simulink model "BFE_TestHarness"  (Simulink 8.6)
settings: Solver=FixedStepDiscrete  StartTime=0.0  StopTime=3  FixedStep=Ts  RelTol=1e-3
PreLoadFcn:
  | addpath('MBD_Tests')
  | 
  | load('Workspace\EnvVar.mat')
  | run('MBD_Tests\MBD_tests_init.m')
  | if exist('tl_preloadfcn','file'), tl_preloadfcn(gcs,402); end
PostLoadFcn:
  | if exist('tl_postloadfcn','file'), tl_postloadfcn(gcs,402); end
InitFcn:
  | if exist('tlds_init','file'), tlds_init(gcs); end
StartFcn:
  | if exist('tlds_start','file'), tlds_start(gcs); end
StopFcn:
  | if exist('tlds_stop','file'), tlds_stop(gcs); end
undefined symbols (not defined in the file): ddv, Ts, u2, u3, u4
libraries: tllib x11, simulink x8, LIB_TF_G_111 x2, LIB_TF_G_12_StepControl x2, LIB_TF_G_112 x1, LIB_TF_G_113 x1
(part 5 of 17)

== system BFE_TestHarness/BFE_AC_BeltFunctionExecution/Subsystem/BFE_AC_BeltFunctionExecution/BFE_AC_BeltFunctionExecution/ManageRunnables/If Action Subsystem2 ==
  PyroTriggeringStatus : Inport
  Trigger : TriggerPort  RequirementInfo={} %GIDa_866c371e_c2ef_4c5d_87b4_f06b2642b18c  TriggerType=function-call
  Constant : Constant  Value=170  mask(TL_Constant){data={'date',735951.66842896992}}
      settings: CopyFcn=if exist('tl_reset_reviewflag','file')==2,tl_reset_reviewflag(gcbh);end  DeleteFcn=if exist('delete_tlblock','file')==2,delete_tlblock(gcbh);end  NameChangeFcn=if exist('rename_tlblock','file')==2,rename_tlblock(gcbh);end  OpenFcn=if exist('tl_open_blockdlg','file')==2,tl_open_blockdlg(gcbh);else,open_system(gcbh,'parameter');end
      mask Help: eval(['if exist(''tl_online_help'',''file'') == 2, tl_online_help(''Topic'',''TL_Constant''),else, web([''jar:file:///'',matlabroot,''/help/toolbox/simulink/help.jar!/slref/' lower(get_param(gcbh,'Blocktype')) '.html''], ''-helpbrowser''),end'])
      mask Display: plot([-0.05, 1.05, NaN, -0.05, 1.05],[.01, .01, NaN, .99, .99])
  If Action Subsystem1 : Subsystem  RequirementInfo={} %GIDa_110f901d_19b3_4a41_884d_c39130871650  TreatAsAtomicUnit=on
  If Action Subsystem2 : Subsystem  RequirementInfo={} %GIDa_d22d9cd8_625f_49e4_bcfa_14ccc98dd57b  TreatAsAtomicUnit=on
  If1 : If  RequirementInfo={} %GIDa_090323af_991c_4502_8351_d7e3f5c13a0a  IfExpression=u1
  Relational Operator : RelationalOperator  Operator===  OutDataTypeStr=boolean  mask(TL_RelationalOperator){data={'date',735951.66842861113}}
      settings: DeleteFcn=if exist('delete_tlblock','file')==2,delete_tlblock(gcbh);end  NameChangeFcn=if exist('rename_tlblock','file')==2,rename_tlblock(gcbh);end  OpenFcn=if exist('tl_open_blockdlg','file')==2,tl_open_blockdlg(gcbh);else,open_system(gcbh,'parameter');end
      mask Help: eval(['if exist(''tl_online_help'',''file'') == 2, tl_online_help(''Topic'',''TL_RelationalOperator''),else, web([''jar:file:///'',matlabroot,''/help/toolbox/simulink/help.jar!/slref/' lower(get_param(gcbh,'Blocktype')) '.html''], ''-helpbrowser''),end'])
      mask Display: plot([-0.05, 1.05, NaN, -0.05, 1.05],[.01, .01, NaN, .99, .99])
  Out1 : Outport  RequirementInfo={} %GIDa_56619d25_d3d5_4dfa_b3ef_d6aa2f335483
  Out2 : Outport  RequirementInfo={} %GIDa_b3d42cdd_db79_4247_be88_47ad93015c12  Port=2
  wires:
  PyroTriggeringStatus/1 -> Relational Operator/2
  Constant/1 -> Relational Operator/1
  Relational Operator/1 -> If1/1
  If1/1 -> If Action Subsystem1/Action
  If Action Subsystem1/1(Out1) -> Out1/1
  If Action Subsystem2/1(Out1) -> Out2/1
  If1/2 -> If Action Subsystem2/Action

== system BFE_TestHarness/BFE_AC_BeltFunctionExecution/Subsystem/BFE_AC_BeltFunctionExecution/BFE_AC_BeltFunctionExecution/ManageRunnables/If Action Subsystem3 ==
  ResetMotorStageStatusRq : Inport
  Trigger : TriggerPort  RequirementInfo={} %GIDa_ecae3cd9_2f7e_4015_a246_5be66d2a3606  TriggerType=function-call
  Constant : Constant  Value=170  mask(TL_Constant){data={'date',735951.66842896992}}
      settings: CopyFcn=if exist('tl_reset_reviewflag','file')==2,tl_reset_reviewflag(gcbh);end  DeleteFcn=if exist('delete_tlblock','file')==2,delete_tlblock(gcbh);end  NameChangeFcn=if exist('rename_tlblock','file')==2,rename_tlblock(gcbh);end  OpenFcn=if exist('tl_open_blockdlg','file')==2,tl_open_blockdlg(gcbh);else,open_system(gcbh,'parameter');end
      mask Help: eval(['if exist(''tl_online_help'',''file'') == 2, tl_online_help(''Topic'',''TL_Constant''),else, web([''jar:file:///'',matlabroot,''/help/toolbox/simulink/help.jar!/slref/' lower(get_param(gcbh,'Blocktype')) '.html''], ''-helpbrowser''),end'])
      mask Display: plot([-0.05, 1.05, NaN, -0.05, 1.05],[.01, .01, NaN, .99, .99])
  If Action Subsystem1 : Subsystem  RequirementInfo={} %GIDa_dd934f85_730c_418a_8463_9eeb7f8d679a  TreatAsAtomicUnit=on
  If1 : If  RequirementInfo={} %GIDa_46faa83a_ad1e_4bf6_b8ac_9d2c86ced2b9  IfExpression=u1  ShowElse=off
  Relational Operator : RelationalOperator  Operator===  OutDataTypeStr=boolean  mask(TL_RelationalOperator){data={'date',735951.66842861113}}
      settings: DeleteFcn=if exist('delete_tlblock','file')==2,delete_tlblock(gcbh);end  NameChangeFcn=if exist('rename_tlblock','file')==2,rename_tlblock(gcbh);end  OpenFcn=if exist('tl_open_blockdlg','file')==2,tl_open_blockdlg(gcbh);else,open_system(gcbh,'parameter');end
      mask Help: eval(['if exist(''tl_online_help'',''file'') == 2, tl_online_help(''Topic'',''TL_RelationalOperator''),else, web([''jar:file:///'',matlabroot,''/help/toolbox/simulink/help.jar!/slref/' lower(get_param(gcbh,'Blocktype')) '.html''], ''-helpbrowser''),end'])
      mask Display: plot([-0.05, 1.05, NaN, -0.05, 1.05],[.01, .01, NaN, .99, .99])
  Out1 : Outport  RequirementInfo={} %GIDa_28cc5c12_1c46_425e_8111_f45bb80ffe30
  wires:
  ResetMotorStageStatusRq/1 -> Relational Operator/2
  Constant/1 -> Relational Operator/1
  Relational Operator/1 -> If1/1
  If1/1 -> If Action Subsystem1/Action
  If Action Subsystem1/1(Out1) -> Out1/1

== system BFE_TestHarness/BFE_AC_BeltFunctionExecution/Subsystem/BFE_AC_BeltFunctionExecution/BFE_AC_BeltFunctionExecution/BFE_runExecuteEmergencyBrakingSequence/ANG regulation/If Action Subsystem1 ==
  MotorPowerOrder : Inport  RequirementInfo={} %GIDa_36d63cdb_a1d7_45a0_bcbf_80961496797e  OutDataTypeStr=int16
  BoostPowerOrder : Inport  RequirementInfo={} %GIDa_d004899a_d052_4335_b4bf_8a07050271f2  Port=2  OutDataTypeStr=int16
  Action Port : ActionPort  RequirementInfo={} %GIDa_6a1bd9e6_01e7_4561_9119_4cca6ef02b4f  ActionType=then
  Data Store Write1 : DataStoreWrite  RequirementInfo={} %GIDa_807db9b2_3118_4ee1_b27d_6a192b350bd3  DataStoreName=BoostPowerOrder  mask(TL_DataStoreWrite){data={'date',735951.66861781245}}
      settings: DeleteFcn=if exist('delete_tlblock','file')==2,delete_tlblock(gcbh);end  NameChangeFcn=if exist('rename_tlblock','file')==2,rename_tlblock(gcbh);end  OpenFcn=if exist('tl_open_blockdlg','file')==2,tl_open_blockdlg(gcbh);else,open_system(gcbh,'parameter');end
      mask Help: eval(['if exist(''tl_online_help'',''file'') == 2, tl_online_help(''Topic'',''TL_DataStoreWrite''),else, web([''jar:file:///'',matlabroot,''/help/toolbox/simulink/help.jar!/slref/' lower(get_param(gcbh,'Blocktype')) '.html''], ''-helpbrowser''),end'])
      mask Display: plot([-0.05, 1.05, NaN, -0.05, 1.05],[.01, .01, NaN, .99, .99])
  Data Store Write2 : DataStoreWrite  RequirementInfo={} %GIDa_2a3ecfdf_d14c_4a9d_9b7c_c5a49fc3f0a5  DataStoreName=MotorPowerOrder  mask(TL_DataStoreWrite){data={'date',735951.6686177199}}
      settings: DeleteFcn=if exist('delete_tlblock','file')==2,delete_tlblock(gcbh);end  NameChangeFcn=if exist('rename_tlblock','file')==2,rename_tlblock(gcbh);end  OpenFcn=if exist('tl_open_blockdlg','file')==2,tl_open_blockdlg(gcbh);else,open_system(gcbh,'parameter');end
      mask Help: eval(['if exist(''tl_online_help'',''file'') == 2, tl_online_help(''Topic'',''TL_DataStoreWrite''),else, web([''jar:file:///'',matlabroot,''/help/toolbox/simulink/help.jar!/slref/' lower(get_param(gcbh,'Blocktype')) '.html''], ''-helpbrowser''),end'])
      mask Display: plot([-0.05, 1.05, NaN, -0.05, 1.05],[.01, .01, NaN, .99, .99])
  wires:
  MotorPowerOrder/1 -> Data Store Write2/1
  BoostPowerOrder/1 -> Data Store Write1/1

== system BFE_TestHarness/BFE_AC_BeltFunctionExecution/Subsystem/BFE_AC_BeltFunctionExecution/BFE_AC_BeltFunctionExecution/BFE_runExecuteEmergencyBrakingSequence/ANG regulation/Product ==
  In_1 : Inport
  In_2 : Inport  Port=2
  In_3 : Inport  Port=3
  Product : Product  Inputs=**  OutDataTypeStr=uint32  RndMeth=Zero  mask(TL_Product){data={'output',{'type','UInt32'},'date',735951.6686142477}}
      settings: CopyFcn=if exist('tl_reset_reviewflag','file')==2,tl_reset_reviewflag(gcbh);end  DeleteFcn=if exist('delete_tlblock','file')==2,delete_tlblock(gcbh);end  NameChangeFcn=if exist('rename_tlblock','file')==2,rename_tlblock(gcbh);end  OpenFcn=if exist('tl_open_blockdlg','file')==2,tl_open_blockdlg(gcbh);else,open_system(gcbh,'parameter');end
      mask Help: eval(['if exist(''tl_online_help'',''file'') == 2, tl_online_help(''Topic'',''TL_Product''),else, web([''jar:file:///'',matlabroot,''/help/toolbox/simulink/help.jar!/slref/' lower(get_param(gcbh,'Blocktype')) '.html''], ''-helpbrowser''),end'])
      mask Display: plot([-0.05, 1.05, NaN, -0.05, 1.05],[.01, .01, NaN, .99, .99])
  Product_1 : Product  Inputs=**  RndMeth=Zero  mask(TL_Product){data={'output',{'type','UInt32'},'date',735951.66861386574}}
      settings: CopyFcn=if exist('tl_reset_reviewflag','file')==2,tl_reset_reviewflag(gcbh);end  DeleteFcn=if exist('delete_tlblock','file')==2,delete_tlblock(gcbh);end  NameChangeFcn=if exist('rename_tlblock','file')==2,rename_tlblock(gcbh);end  OpenFcn=if exist('tl_open_blockdlg','file')==2,tl_open_blockdlg(gcbh);else,open_system(gcbh,'parameter');end
      mask Help: eval(['if exist(''tl_online_help'',''file'') == 2, tl_online_help(''Topic'',''TL_Product''),else, web([''jar:file:///'',matlabroot,''/help/toolbox/simulink/help.jar!/slref/' lower(get_param(gcbh,'Blocktype')) '.html''], ''-helpbrowser''),end'])
      mask Display: plot([-0.05, 1.05, NaN, -0.05, 1.05],[.01, .01, NaN, .99, .99])
  Out_1 : Outport
  wires:
  In_1/1 -> Product_1/1
  In_2/1 -> Product_1/2
  In_3/1 -> Product/2
  Product_1/1 -> Product/1
  Product/1 -> Out_1/1

== system BFE_TestHarness/BFE_AC_BeltFunctionExecution/Subsystem/BFE_AC_BeltFunctionExecution/BFE_AC_BeltFunctionExecution/BFE_runExecuteEmergencyBrakingSequence/ANG regulation/Src ==
  Const : Constant  Value=ddv('RTE_Define/KU8_MOTOR_STAGE_EMERGENCY_DEACTIVATION')  mask(TL_Constant){data={'output',{'variable','RTE_Define/KU8_MOTOR_STAGE_EMERGENCY_DEACTIVATION'},'date',735951.66861100693}}
      settings: CopyFcn=if exist('tl_reset_reviewflag','file')==2,tl_reset_reviewflag(gcbh);end  DeleteFcn=if exist('delete_tlblock','file')==2,delete_tlblock(gcbh);end  NameChangeFcn=if exist('rename_tlblock','file')==2,rename_tlblock(gcbh);end  OpenFcn=if exist('tl_open_blockdlg','file')==2,tl_open_blockdlg(gcbh);else,open_system(gcbh,'parameter');end
      mask Help: eval(['if exist(''tl_online_help'',''file'') == 2, tl_online_help(''Topic'',''TL_Constant''),else, web([''jar:file:///'',matlabroot,''/help/toolbox/simulink/help.jar!/slref/' lower(get_param(gcbh,'Blocktype')) '.html''], ''-helpbrowser''),end'])
      mask Display: plot([-0.05, 1.05, NaN, -0.05, 1.05],[.01, .01, NaN, .99, .99])
  u8MotorStageStatus : Outport
  wires:
  Const/1 -> u8MotorStageStatus/1  "u8MotorStageStatus"

== system BFE_TestHarness/BFE_AC_BeltFunctionExecution/Subsystem/BFE_AC_BeltFunctionExecution/BFE_AC_BeltFunctionExecution/BFE_runExecuteEmergencyBrakingSequence/Idle State/If Action Subsystem ==
  MotorPowerOrder : Inport  RequirementInfo={} %GIDa_39707416_cbd7_49a4_89b1_309ad3050f45  OutDataTypeStr=int16
  BoostPowerOrder : Inport  RequirementInfo={} %GIDa_de3b3d4e_919a_4afc_a9bd_d52a78375d81  Port=2  OutDataTypeStr=int16
  Action Port : ActionPort  RequirementInfo={} %GIDa_e9528953_7f61_49b7_b615_23fe905f704f  ActionType=then
  Data Store Write1 : DataStoreWrite  RequirementInfo={} %GIDa_59c6ee34_e957_4309_9132_375d2670ef26  DataStoreName=BoostPowerOrder  mask(TL_DataStoreWrite){data={'date',735951.66860575229}}
      settings: DeleteFcn=if exist('delete_tlblock','file')==2,delete_tlblock(gcbh);end  NameChangeFcn=if exist('rename_tlblock','file')==2,rename_tlblock(gcbh);end  OpenFcn=if exist('tl_open_blockdlg','file')==2,tl_open_blockdlg(gcbh);else,open_system(gcbh,'parameter');end
      mask Help: eval(['if exist(''tl_online_help'',''file'') == 2, tl_online_help(''Topic'',''TL_DataStoreWrite''),else, web([''jar:file:///'',matlabroot,''/help/toolbox/simulink/help.jar!/slref/' lower(get_param(gcbh,'Blocktype')) '.html''], ''-helpbrowser''),end'])
      mask Display: plot([-0.05, 1.05, NaN, -0.05, 1.05],[.01, .01, NaN, .99, .99])
  Data Store Write2 : DataStoreWrite  RequirementInfo={} %GIDa_3b8346d3_29b2_4ee4_8164_42224b922a82  DataStoreName=MotorPowerOrder  mask(TL_DataStoreWrite){data={'date',735951.6686056481}}
      settings: DeleteFcn=if exist('delete_tlblock','file')==2,delete_tlblock(gcbh);end  NameChangeFcn=if exist('rename_tlblock','file')==2,rename_tlblock(gcbh);end  OpenFcn=if exist('tl_open_blockdlg','file')==2,tl_open_blockdlg(gcbh);else,open_system(gcbh,'parameter');end
      mask Help: eval(['if exist(''tl_online_help'',''file'') == 2, tl_online_help(''Topic'',''TL_DataStoreWrite''),else, web([''jar:file:///'',matlabroot,''/help/toolbox/simulink/help.jar!/slref/' lower(get_param(gcbh,'Blocktype')) '.html''], ''-helpbrowser''),end'])
      mask Display: plot([-0.05, 1.05, NaN, -0.05, 1.05],[.01, .01, NaN, .99, .99])
  wires:
  MotorPowerOrder/1 -> Data Store Write2/1
  BoostPowerOrder/1 -> Data Store Write1/1

== system BFE_TestHarness/BFE_AC_BeltFunctionExecution/Subsystem/BFE_AC_BeltFunctionExecution/BFE_AC_BeltFunctionExecution/BFE_runExecuteEmergencyBrakingSequence/Idle State/Src ==
  Const : Constant  Value=ddv('RTE_Define/KU8_MOTOR_STAGE_EMERGENCY_DEACTIVATION')  mask(TL_Constant){data={'output',{'variable','RTE_Define/KU8_MOTOR_STAGE_EMERGENCY_DEACTIVATION'},'date',735951.66860392364}}
      settings: CopyFcn=if exist('tl_reset_reviewflag','file')==2,tl_reset_reviewflag(gcbh);end  DeleteFcn=if exist('delete_tlblock','file')==2,delete_tlblock(gcbh);end  NameChangeFcn=if exist('rename_tlblock','file')==2,rename_tlblock(gcbh);end  OpenFcn=if exist('tl_open_blockdlg','file')==2,tl_open_blockdlg(gcbh);else,open_system(gcbh,'parameter');end
      mask Help: eval(['if exist(''tl_online_help'',''file'') == 2, tl_online_help(''Topic'',''TL_Constant''),else, web([''jar:file:///'',matlabroot,''/help/toolbox/simulink/help.jar!/slref/' lower(get_param(gcbh,'Blocktype')) '.html''], ''-helpbrowser''),end'])
      mask Display: plot([-0.05, 1.05, NaN, -0.05, 1.05],[.01, .01, NaN, .99, .99])
  u8MotorStageStatus : Outport
  wires:
  Const/1 -> u8MotorStageStatus/1  "u8MotorStageStatus"

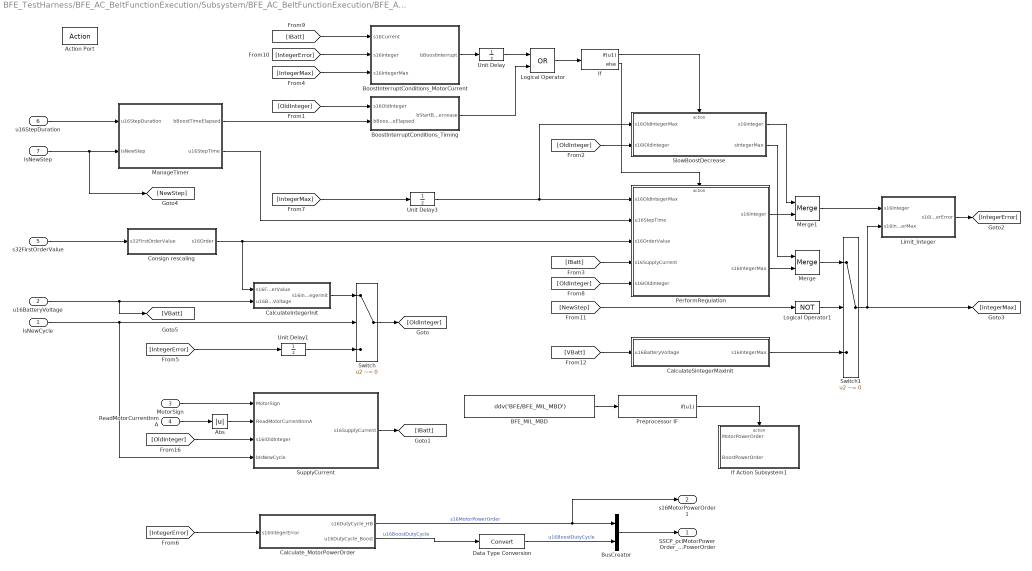
== system BFE_TestHarness/BFE_AC_BeltFunctionExecution/Subsystem/BFE_AC_BeltFunctionExecution/BFE_AC_BeltFunctionExecution/BFE_runExecuteHighPowerStep/HP feature activated/CurrentRegulation ==
  IsNewCycle : Inport  RequirementInfo={} %GIDa_1662e31c_4847_435c_863a_1ec5eca2756d
  u16BatteryVoltage : Inport  RequirementInfo={} %GIDa_1bb34935_6dbf_432a_9b43_0281e74792fd  Port=2
  MotorSign : Inport  RequirementInfo={} %GIDa_5fb47f80_c22b_46b0_b1d3_660182323a24  Port=3
  ReadMotorCurrentInmA : Inport  RequirementInfo={} %GIDa_31f7513d_9132_45be_9a79_4368bb0828a9  Port=4
  s32FirstOrderValue : Inport  RequirementInfo={} %GIDa_e04d25b8_d427_4e8e_8f00_3b1e8e5fec68  Port=5
  u16StepDuration : Inport  RequirementInfo={} %GIDa_4dbadef5_81a2_48d0_a2ca_74b2fd0262db  Port=6  OutDataTypeStr=uint16
  IsNewStep : Inport  RequirementInfo={} %GIDa_223ba4e3_ba54_41a4_96d0_22f7bdf9d99f  Port=7
  Action Port : ActionPort  RequirementInfo={} %GIDa_dfa5435c_c4b1_4a26_8b12_c66635d4e3dc  ActionType=then
  Abs : Abs  mask(TL_Abs){data={'output',{'type','UInt32'},'date',735951.66858795134}}
      settings: CopyFcn=if exist('tl_reset_reviewflag','file')==2,tl_reset_reviewflag(gcbh);end  DeleteFcn=if exist('delete_tlblock','file')==2,delete_tlblock(gcbh);end  NameChangeFcn=if exist('rename_tlblock','file')==2,rename_tlblock(gcbh);end  OpenFcn=if exist('tl_open_blockdlg','file')==2,tl_open_blockdlg(gcbh);else,open_system(gcbh,'parameter');end
      mask Help: eval(['if exist(''tl_online_help'',''file'') == 2, tl_online_help(''Topic'',''TL_Abs''),else, web([''jar:file:///'',matlabroot,''/help/toolbox/simulink/help.jar!/slref/' lower(get_param(gcbh,'Blocktype')) '.html''], ''-helpbrowser''),end'])
      mask Display: plot([-0.05, 1.05, NaN, -0.05, 1.05],[.01, .01, NaN, .99, .99])
  BFE_MIL_MBD : Constant  RequirementInfo={} %GIDa_b0161e3c_e162_4059_a91d_45f997bd6b1e  Value=ddv('BFE/BFE_MIL_MBD')  mask(TL_Constant){data={'output',{'variable','BFE/BFE_MIL_MBD'},'date',735951.66858758102}}
      settings: CopyFcn=if exist('tl_reset_reviewflag','file')==2,tl_reset_reviewflag(gcbh);end  DeleteFcn=if exist('delete_tlblock','file')==2,delete_tlblock(gcbh);end  NameChangeFcn=if exist('rename_tlblock','file')==2,rename_tlblock(gcbh);end  OpenFcn=if exist('tl_open_blockdlg','file')==2,tl_open_blockdlg(gcbh);else,open_system(gcbh,'parameter');end
      mask Help: eval(['if exist(''tl_online_help'',''file'') == 2, tl_online_help(''Topic'',''TL_Constant''),else, web([''jar:file:///'',matlabroot,''/help/toolbox/simulink/help.jar!/slref/' lower(get_param(gcbh,'Blocktype')) '.html''], ''-helpbrowser''),end'])
      mask Display: plot([-0.05, 1.05, NaN, -0.05, 1.05],[.01, .01, NaN, .99, .99])
  BoostInterruptConditions_MotorCurrent : Subsystem  RequirementInfo={} %GIDa_1e154413_408a_4156_80c5_1742329dab2b
  BoostInterruptConditions_Timing : Subsystem  RequirementInfo={} %GIDa_8282939d_02dc_455b_ba62_25a73597f55d
  BusCreator : BusCreator  Inputs=2
  CalculateIntegerInit : Subsystem  RequirementInfo={} %GIDa_9a2c8a86_eea1_4d27_b0ce_971bbb33bd14
  CalculateSintegerMaxInit : Subsystem  RequirementInfo={} %GIDa_66e9dbb1_52b6_4aae_afa6_381740208472  TreatAsAtomicUnit=on
  Calculate_MotorPowerOrder : Subsystem  RequirementInfo={} %GIDa_f695fff8_9d75_4e11_9ea4_5644486dca77
  Consign rescaling : Subsystem  TreatAsAtomicUnit=on
      settings: AttributesFormatString=8092 lsb = 0.5 [A]\nV\n1 lsb = 10 [mA]
  Data Type Conversion : DataTypeConversion
  If : If  RequirementInfo={} %GIDa_93686889_67cf_4afb_8e2f_6a5e4d238abf  IfExpression=u1
  If Action Subsystem1 : Subsystem  RequirementInfo={} %GIDa_73714641_df61_49fe_9fdd_bd97cd5bece8  TreatAsAtomicUnit=on
  Limit_Integer : Subsystem  RequirementInfo={} %GIDa_70b31615_98db_428c_aa79_8c8fa2e5a701
  Logical Operator : Logic  RequirementInfo={} %GIDa_fe6e0a6b_febe_46e6_a7cb_d3961de08f42  Operator=OR  AllPortsSameDT=off  OutDataTypeStr=boolean  mask(TL_LogicalOperator){data={'date',735951.66856991895}}
      settings: DeleteFcn=if exist('delete_tlblock','file')==2,delete_tlblock(gcbh);end  NameChangeFcn=if exist('rename_tlblock','file')==2,rename_tlblock(gcbh);end  OpenFcn=if exist('tl_open_blockdlg','file')==2,tl_open_blockdlg(gcbh);else,open_system(gcbh,'parameter');end
      mask Help: eval(['if exist(''tl_online_help'',''file'') == 2, tl_online_help(''Topic'',''TL_LogicalOperator''),else, web([''jar:file:///'',matlabroot,''/help/toolbox/simulink/help.jar!/slref/' lower(get_param(gcbh,'Blocktype')) '.html''], ''-helpbrowser''),end'])
      mask Display: plot([-0.05, 1.05, NaN, -0.05, 1.05],[.01, .01, NaN, .99, .99])
  Logical Operator1 : Logic  Operator=NOT  Inputs=1  AllPortsSameDT=off  OutDataTypeStr=boolean  mask(TL_LogicalOperator){data={'date',735951.66856965283}}
      settings: DeleteFcn=if exist('delete_tlblock','file')==2,delete_tlblock(gcbh);end  NameChangeFcn=if exist('rename_tlblock','file')==2,rename_tlblock(gcbh);end  OpenFcn=if exist('tl_open_blockdlg','file')==2,tl_open_blockdlg(gcbh);else,open_system(gcbh,'parameter');end
      mask Help: eval(['if exist(''tl_online_help'',''file'') == 2, tl_online_help(''Topic'',''TL_LogicalOperator''),else, web([''jar:file:///'',matlabroot,''/help/toolbox/simulink/help.jar!/slref/' lower(get_param(gcbh,'Blocktype')) '.html''], ''-helpbrowser''),end'])
      mask Display: plot([-0.05, 1.05, NaN, -0.05, 1.05],[.01, .01, NaN, .99, .99])
  ManageTimer : Subsystem  RequirementInfo={} %GIDa_aa7b4bf5_2b52_4aaf_8bb3_ae9b1da1e681
  Merge : Merge  RequirementInfo={} %GIDa_abd3f291_8f58_447c_99f5_868d95eb83d7  InitialOutput=0  mask(TL_Merge){data={'output',{'name','s16IntegerMaxOnGoing'},'date',735951.66844865738}}
      settings: CopyFcn=if exist('tl_reset_reviewflag','file')==2,tl_reset_reviewflag(gcbh);end  DeleteFcn=if exist('delete_tlblock','file')==2,delete_tlblock(gcbh);end  NameChangeFcn=if exist('rename_tlblock','file')==2,rename_tlblock(gcbh);end  OpenFcn=if exist('tl_open_blockdlg','file')==2,tl_open_blockdlg(gcbh);else,open_system(gcbh,'parameter');end
      mask Help: eval(['if exist(''tl_online_help'',''file'') == 2, tl_online_help(''Topic'',''TL_Merge''),else, web([''jar:file:///'',matlabroot,''/help/toolbox/simulink/help.jar!/slref/' lower(get_param(gcbh,'Blocktype')) '.html''], ''-helpbrowser''),end'])
      mask Display: plot([-0.05, 1.05, NaN, -0.05, 1.05],[.01, .01, NaN, .99, .99])
  Merge1 : Merge  RequirementInfo={} %GIDa_8234cb0a_dc3c_4713_a3c9_c2ddd3d4af5c  InitialOutput=0  mask(TL_Merge){data={'output',{'name','s16Integer'},'date',735951.66844827542}}
      settings: CopyFcn=if exist('tl_reset_reviewflag','file')==2,tl_reset_reviewflag(gcbh);end  DeleteFcn=if exist('delete_tlblock','file')==2,delete_tlblock(gcbh);end  NameChangeFcn=if exist('rename_tlblock','file')==2,rename_tlblock(gcbh);end  OpenFcn=if exist('tl_open_blockdlg','file')==2,tl_open_blockdlg(gcbh);else,open_system(gcbh,'parameter');end
      mask Help: eval(['if exist(''tl_online_help'',''file'') == 2, tl_online_help(''Topic'',''TL_Merge''),else, web([''jar:file:///'',matlabroot,''/help/toolbox/simulink/help.jar!/slref/' lower(get_param(gcbh,'Blocktype')) '.html''], ''-helpbrowser''),end'])
      mask Display: plot([-0.05, 1.05, NaN, -0.05, 1.05],[.01, .01, NaN, .99, .99])
  PerformRegulation : Subsystem  RequirementInfo={} %GIDa_1363a116_a98c_4e77_a913_b87844d45823
  Preprocessor IF : If  RequirementInfo={} %GIDa_f50148b4_caa7_4fb8_ad64_c4c8bcffd358  IfExpression=u1  ShowElse=off  mask(TL_PreProcessorIf){data={'mode',2,'date',735951.66844163195}}
      settings: DeleteFcn=if exist('delete_tlblock','file')==2,delete_tlblock(gcbh);end  NameChangeFcn=if exist('rename_tlblock','file')==2,rename_tlblock(gcbh);end  OpenFcn=if exist('tl_open_blockdlg','file')==2,tl_open_blockdlg(gcbh);else,open_system(gcbh,'parameter');end
      mask Help: eval(['if exist(''tl_online_help'',''file'') == 2, tl_online_help(''Topic'',''TL_PreProcessorIf''),else, web([''jar:file:///'',matlabroot,''/help/toolbox/simulink/help.jar!/slref/' lower(get_param(gcbh,'Blocktype')) '.html''], ''-helpbrowser''),end'])
      mask Display:
      | plot([-0.05, 1.05, NaN, -0.05, 1.05],[.01, .01, NaN, .99, .99])
      | 
      | port_label('input', 1, 'u1')
      | port_label('output',1,'#ifdef u1');
  SlowBoostDecrease : Subsystem  RequirementInfo={} %GIDa_3dda9a5c_4141_4318_8fb6_6c48e8effe73
  SupplyCurrent : Subsystem  TreatAsAtomicUnit=on
  Switch : Switch  RequirementInfo={} %GIDa_30553cb4_fd4d_48f0_a467_0ca3f5a035ff  Criteria=u2 ~= 0  mask(TL_Switch){data={'output',{'name','s16OldIntegerError'},'date',735951.66841892363}}
      settings: CopyFcn=if exist('tl_reset_reviewflag','file')==2,tl_reset_reviewflag(gcbh);end  DeleteFcn=if exist('delete_tlblock','file')==2,delete_tlblock(gcbh);end  NameChangeFcn=if exist('rename_tlblock','file')==2,rename_tlblock(gcbh);end  OpenFcn=if exist('tl_open_blockdlg','file')==2,tl_open_blockdlg(gcbh);else,open_system(gcbh,'parameter');end
      mask Help: eval(['if exist(''tl_online_help'',''file'') == 2, tl_online_help(''Topic'',''TL_Switch''),else, web([''jar:file:///'',matlabroot,''/help/toolbox/simulink/help.jar!/slref/' lower(get_param(gcbh,'Blocktype')) '.html''], ''-helpbrowser''),end'])
      mask Display: plot([-0.05, 1.05, NaN, -0.05, 1.05],[.01, .01, NaN, .99, .99])
  Switch1 : Switch  Criteria=u2 ~= 0  mask(TL_Switch){data={'output',{'name','s16IntegerMax'},'date',735951.66841839126}}
      settings: CopyFcn=if exist('tl_reset_reviewflag','file')==2,tl_reset_reviewflag(gcbh);end  DeleteFcn=if exist('delete_tlblock','file')==2,delete_tlblock(gcbh);end  NameChangeFcn=if exist('rename_tlblock','file')==2,rename_tlblock(gcbh);end  OpenFcn=if exist('tl_open_blockdlg','file')==2,tl_open_blockdlg(gcbh);else,open_system(gcbh,'parameter');end
      mask Help: eval(['if exist(''tl_online_help'',''file'') == 2, tl_online_help(''Topic'',''TL_Switch''),else, web([''jar:file:///'',matlabroot,''/help/toolbox/simulink/help.jar!/slref/' lower(get_param(gcbh,'Blocktype')) '.html''], ''-helpbrowser''),end'])
      mask Display: plot([-0.05, 1.05, NaN, -0.05, 1.05],[.01, .01, NaN, .99, .99])
  Unit Delay : UnitDelay  RequirementInfo={} %GIDa_40b8b31e_7c77_49f4_a8c4_1aef21ac2334  SampleTime=-1  mask(TL_UnitDelay){data={'state',{'name','bOldBoostInterrupt'},'date',735951.66841787042}}
      settings: CopyFcn=if exist('tl_reset_reviewflag','file')==2,tl_reset_reviewflag(gcbh);end  DeleteFcn=if exist('delete_tlblock','file')==2,delete_tlblock(gcbh);end  NameChangeFcn=if exist('rename_tlblock','file')==2,rename_tlblock(gcbh);end  OpenFcn=if exist('tl_open_blockdlg','file')==2,tl_open_blockdlg(gcbh);else,open_system(gcbh,'parameter');end
      mask Help: eval(['if exist(''tl_online_help'',''file'') == 2, tl_online_help(''Topic'',''TL_UnitDelay''),else, web([''jar:file:///'',matlabroot,''/help/toolbox/simulink/help.jar!/slref/' lower(get_param(gcbh,'Blocktype')) '.html''], ''-helpbrowser''),end'])
      mask Display: plot([-0.05, 1.05, NaN, -0.05, 1.05],[.01, .01, NaN, .99, .99])
  Unit Delay1 : UnitDelay  RequirementInfo={} %GIDa_fff37aa9_a0a1_4cec_b06f_6507d85e68da  SampleTime=-1  mask(TL_UnitDelay){data={'state',{'name','s16_OldIntegerError'},'date',735951.66841733793}}
      settings: CopyFcn=if exist('tl_reset_reviewflag','file')==2,tl_reset_reviewflag(gcbh);end  DeleteFcn=if exist('delete_tlblock','file')==2,delete_tlblock(gcbh);end  NameChangeFcn=if exist('rename_tlblock','file')==2,rename_tlblock(gcbh);end  OpenFcn=if exist('tl_open_blockdlg','file')==2,tl_open_blockdlg(gcbh);else,open_system(gcbh,'parameter');end
      mask Help: eval(['if exist(''tl_online_help'',''file'') == 2, tl_online_help(''Topic'',''TL_UnitDelay''),else, web([''jar:file:///'',matlabroot,''/help/toolbox/simulink/help.jar!/slref/' lower(get_param(gcbh,'Blocktype')) '.html''], ''-helpbrowser''),end'])
      mask Display: plot([-0.05, 1.05, NaN, -0.05, 1.05],[.01, .01, NaN, .99, .99])
  Unit Delay3 : UnitDelay  RequirementInfo={} %GIDa_408d93ed_0585_4d91_8b20_90bf83d81e20  SampleTime=-1  mask(TL_UnitDelay){data={'state',{'name','s16OldIntegerMax'},'date',735951.66841681709}}
      settings: CopyFcn=if exist('tl_reset_reviewflag','file')==2,tl_reset_reviewflag(gcbh);end  DeleteFcn=if exist('delete_tlblock','file')==2,delete_tlblock(gcbh);end  NameChangeFcn=if exist('rename_tlblock','file')==2,rename_tlblock(gcbh);end  OpenFcn=if exist('tl_open_blockdlg','file')==2,tl_open_blockdlg(gcbh);else,open_system(gcbh,'parameter');end
      mask Help: eval(['if exist(''tl_online_help'',''file'') == 2, tl_online_help(''Topic'',''TL_UnitDelay''),else, web([''jar:file:///'',matlabroot,''/help/toolbox/simulink/help.jar!/slref/' lower(get_param(gcbh,'Blocktype')) '.html''], ''-helpbrowser''),end'])
      mask Display: plot([-0.05, 1.05, NaN, -0.05, 1.05],[.01, .01, NaN, .99, .99])
  SSCP_pclMotorPowerOrder_SetPowerOrder : Outport  mask(TL_BusOutport){data={'#autoscaling',2,'#message',2,'#output',2,'#logdata',2,'signals',{{'',{'s16MotorPowerOrder';'u16BoostDutyCycle'}}},'autosar',{'useautosarcommunication',1,'kind',4,'clientserverport','pclMotor_P','operation','SetPowerOrder'},'date',736301.7172136805}}
      settings: CopyFcn=if exist('tl_reset_reviewflag','file')==2,tl_reset_reviewflag(gcbh);end  DeleteFcn=if exist('delete_tlblock','file')==2,delete_tlblock(gcbh);end  NameChangeFcn=if exist('rename_tlblock','file')==2,rename_tlblock(gcbh);end  OpenFcn=if exist('tl_open_blockdlg','file')==2,tl_open_blockdlg(gcbh);else,open_system(gcbh,'parameter');end
      mask Help: eval(['if exist(''tl_online_help'',''file'') == 2, tl_online_help(''Topic'',''TL_Outport''),else, web([''jar:file:///'',matlabroot,''/help/toolbox/simulink/help.jar!/slref/' lower(get_param(gcbh,'Blocktype')) '.html''], ''-helpbrowser''),end'])
      mask Display: plot([0.2 0.35 NaN 0.65 0.8],[0 1 NaN 0 1]);
  s16MotorPowerOrder1 : Outport  Port=2  PortDimensions=1  InitialOutput=0  mask(TL_Outport){data={'autosar',{'useautosarcommunication',1,'kind',3,'communicationmode',1,'interrunnablevariable','s16MotorPowerOrder'},'date',736809.44014787034}}
      settings: CopyFcn=if exist('tl_reset_reviewflag','file')==2,tl_reset_reviewflag(gcbh);end  DeleteFcn=if exist('delete_tlblock','file')==2,delete_tlblock(gcbh);end  NameChangeFcn=if exist('rename_tlblock','file')==2,rename_tlblock(gcbh);end  OpenFcn=if exist('tl_open_blockdlg','file')==2,tl_open_blockdlg(gcbh);else,open_system(gcbh,'parameter');end
      mask Help: eval(['if exist(''tl_online_help'',''file'') == 2, tl_online_help(''Topic'',''TL_Outport''),else, web([''jar:file:///'',matlabroot,''/help/toolbox/simulink/help.jar!/slref/' lower(get_param(gcbh,'Blocktype')) '.html''], ''-helpbrowser''),end'])
      mask Display: plot([0.2 0.35 NaN 0.65 0.8],[0 1 NaN 0 1]);
  wires:
  If/1 -> SlowBoostDecrease/Action
  If/2 -> PerformRegulation/Action
  s32FirstOrderValue/1 -> Consign rescaling/1(s32FirstOrderValue)
  IsNewStep/1 -> ManageTimer/2(IsNewStep), [NewStep]
  u16StepDuration/1 -> ManageTimer/1(u16StepDuration)
  SlowBoostDecrease/2(sIntegerMax) -> Merge/1
  PerformRegulation/1(s16Integer) -> Merge1/2
  CalculateIntegerInit/1(s16IntegerInit) -> Switch/1
  Unit Delay1/1 -> Switch/3
  SlowBoostDecrease/1(s16Integer) -> Merge1/1
  MotorSign/1 -> SupplyCurrent/1(MotorSign)
  ReadMotorCurrentInmA/1 -> Abs/1
  IsNewCycle/1 -> Switch/2, SupplyCurrent/4(bIsNewCycle)
  Logical Operator/1 -> If/1
  PerformRegulation/2(s16IntegerMax) -> Merge/2
  ManageTimer/1(bBoostTimeElapsed) -> BoostInterruptConditions_Timing/2(bBoostTimeElapsed)
  BoostInterruptConditions_Timing/1(bStartBoostDecrease) -> Logical Operator/2
  Switch/1 -> [OldInteger]
  [OldInteger] -> BoostInterruptConditions_Timing/1(s16OldInteger)
  [OldInteger] -> SlowBoostDecrease/2(s16IOldInteger)
  Unit Delay/1 -> Logical Operator/1
  SupplyCurrent/1(s16SupplyCurrent) -> [IBatt]
  [IBatt] -> PerformRegulation/4(s16SupplyCurrent)
  [IntegerError] -> Unit Delay1/1
  [OldInteger] -> PerformRegulation/5(s16IOldInteger)
  [IBatt] -> BoostInterruptConditions_MotorCurrent/1(s16Current)
  [IntegerError] -> BoostInterruptConditions_MotorCurrent/2(s16Integer)
  BoostInterruptConditions_MotorCurrent/1(bBoostInterrupt) -> Unit Delay/1
  Consign rescaling/1(s16Order) -> PerformRegulation/3(s16OrderValue), CalculateIntegerInit/1(s16FirstOrderValue)
  Unit Delay3/1 -> SlowBoostDecrease/1(s16OldIntegerMax), PerformRegulation/1(s16OldIntegerMax)
  [IntegerMax] -> BoostInterruptConditions_MotorCurrent/3(s16IntegerMax)
  [IntegerMax] -> Unit Delay3/1
  u16BatteryVoltage/1 -> CalculateIntegerInit/2(u16BatteryVoltage), [VBatt]
  Merge/1 -> Switch1/1
  CalculateSintegerMaxInit/1(s16IntegerMax) -> Switch1/3
  Switch1/1 -> Limit_Integer/2(s16IntegerMax), [IntegerMax]
  [NewStep] -> Logical Operator1/1
  Logical Operator1/1 -> Switch1/2
  [VBatt] -> CalculateSintegerMaxInit/1(u16BatteryVoltage)
  [OldInteger] -> SupplyCurrent/3(s16IOldInteger)
  Calculate_MotorPowerOrder/1(s16DutyCycle_HB) -> BusCreator/1, s16MotorPowerOrder1/1  "s16MotorPowerOrder"
  Calculate_MotorPowerOrder/2(u16DutyCycle_Boost) -> Data Type Conversion/1  "u16BoostDutyCycle"
  BusCreator/1 -> SSCP_pclMotorPowerOrder_SetPowerOrder/1
  ManageTimer/2(u16StepTime) -> PerformRegulation/2(u16StepTime)
  Limit_Integer/1(s16IntegerError) -> [IntegerError]
  Merge1/1 -> Limit_Integer/1(s16Integer)
  [IntegerError] -> Calculate_MotorPowerOrder/1(s16IntegerError)
  Abs/1 -> SupplyCurrent/2(ReadMotorCurrentInmA)
  Preprocessor IF/1 -> If Action Subsystem1/Action
  BFE_MIL_MBD/1 -> Preprocessor IF/1
  Data Type Conversion/1 -> BusCreator/2  "u16BoostDutyCycle"

== system BFE_TestHarness/BFE_AC_BeltFunctionExecution/Subsystem/BFE_AC_BeltFunctionExecution/BFE_AC_BeltFunctionExecution/BFE_runExecuteHighPowerStep/HP feature activated/IsNewCycle ==
  u8OrderType : Inport  RequirementInfo={} %GIDa_93952be5_c99b_45cd_83e0_90b61eb2f782
  KUC_ORDER_NO_STEP : Constant  RequirementInfo={} %GIDa_81993007_4661_4fd9_886f_ede9d0b66024  Value=ddv('BFE/Step_Def/KU8_NO_STEP_TYPE')  mask(TL_Constant){data={'output',{'variable','BFE/Step_Def/KU8_NO_STEP_TYPE'},'date',735951.66841428238}}
      settings: CopyFcn=if exist('tl_reset_reviewflag','file')==2,tl_reset_reviewflag(gcbh);end  DeleteFcn=if exist('delete_tlblock','file')==2,delete_tlblock(gcbh);end  NameChangeFcn=if exist('rename_tlblock','file')==2,rename_tlblock(gcbh);end  OpenFcn=if exist('tl_open_blockdlg','file')==2,tl_open_blockdlg(gcbh);else,open_system(gcbh,'parameter');end
      mask Help: eval(['if exist(''tl_online_help'',''file'') == 2, tl_online_help(''Topic'',''TL_Constant''),else, web([''jar:file:///'',matlabroot,''/help/toolbox/simulink/help.jar!/slref/' lower(get_param(gcbh,'Blocktype')) '.html''], ''-helpbrowser''),end'])
      mask Display: plot([-0.05, 1.05, NaN, -0.05, 1.05],[.01, .01, NaN, .99, .99])
  Relational Operator : RelationalOperator  RequirementInfo={} %GIDa_8d2fc2a3_17b7_4425_80b3_ecb73767892b  Operator===  OutDataTypeStr=boolean  mask(TL_RelationalOperator){data={'output',{'name','bIsNewCycle'},'date',735951.66841391206}}
      settings: DeleteFcn=if exist('delete_tlblock','file')==2,delete_tlblock(gcbh);end  NameChangeFcn=if exist('rename_tlblock','file')==2,rename_tlblock(gcbh);end  OpenFcn=if exist('tl_open_blockdlg','file')==2,tl_open_blockdlg(gcbh);else,open_system(gcbh,'parameter');end
      mask Help: eval(['if exist(''tl_online_help'',''file'') == 2, tl_online_help(''Topic'',''TL_RelationalOperator''),else, web([''jar:file:///'',matlabroot,''/help/toolbox/simulink/help.jar!/slref/' lower(get_param(gcbh,'Blocktype')) '.html''], ''-helpbrowser''),end'])
      mask Display: plot([-0.05, 1.05, NaN, -0.05, 1.05],[.01, .01, NaN, .99, .99])
  Unit Delay2 : UnitDelay  RequirementInfo={} %GIDa_e33fd28c_43c0_41aa_857d_1ac3251269ea  SampleTime=-1  mask(TL_UnitDelay){data={'output',{'type','UInt8'},'state',{'name','u8OldOrderType','type','UInt8'},'date',735951.6684136343}}
      settings: CopyFcn=if exist('tl_reset_reviewflag','file')==2,tl_reset_reviewflag(gcbh);end  DeleteFcn=if exist('delete_tlblock','file')==2,delete_tlblock(gcbh);end  NameChangeFcn=if exist('rename_tlblock','file')==2,rename_tlblock(gcbh);end  OpenFcn=if exist('tl_open_blockdlg','file')==2,tl_open_blockdlg(gcbh);else,open_system(gcbh,'parameter');end
      mask Help: eval(['if exist(''tl_online_help'',''file'') == 2, tl_online_help(''Topic'',''TL_UnitDelay''),else, web([''jar:file:///'',matlabroot,''/help/toolbox/simulink/help.jar!/slref/' lower(get_param(gcbh,'Blocktype')) '.html''], ''-helpbrowser''),end'])
      mask Display: plot([-0.05, 1.05, NaN, -0.05, 1.05],[.01, .01, NaN, .99, .99])
  IsNewCycle : Outport  RequirementInfo={} %GIDa_1e550a25_008c_4c6b_988d_fe4f27871434
  wires:
  u8OrderType/1 -> Unit Delay2/1
  Unit Delay2/1 -> Relational Operator/1
  Relational Operator/1 -> IsNewCycle/1
  KUC_ORDER_NO_STEP/1 -> Relational Operator/2

== system BFE_TestHarness/BFE_AC_BeltFunctionExecution/Subsystem/BFE_AC_BeltFunctionExecution/BFE_AC_BeltFunctionExecution/BFE_runExecuteStandardSteps/ExecuteStandardSteps/Mange Power Stage consign update ==
  u8MotorStageStatus : Inport  PortDimensions=1  mask(TL_Inport){data={'autosar',{'useautosarcommunication',1,'kind',3,'interrunnablevariable','u8MotorStageStatus'},'date',736809.44014868059}}
      settings: CopyFcn=if exist('tl_reset_reviewflag','file')==2,tl_reset_reviewflag(gcbh);end  DeleteFcn=if exist('delete_tlblock','file')==2,delete_tlblock(gcbh);end  NameChangeFcn=if exist('rename_tlblock','file')==2,rename_tlblock(gcbh);end  OpenFcn=if exist('tl_open_blockdlg','file')==2,tl_open_blockdlg(gcbh);else,open_system(gcbh,'parameter');end
      mask Help: eval(['if exist(''tl_online_help'',''file'') == 2, tl_online_help(''Topic'',''TL_Inport''),else, web([''jar:file:///'',matlabroot,''/help/toolbox/simulink/help.jar!/slref/' lower(get_param(gcbh,'Blocktype')) '.html''], ''-helpbrowser''),end'])
      mask Display: plot([0.2 0.35 NaN 0.65 0.8],[0 1 NaN 0 1]);
  In1 : Inport  Port=2
  Call PAL service to update the PWM : Subsystem  TreatAsAtomicUnit=on
  Demux : Demux  Outputs=3
  Function-Call Generator : simulink/Ports & Subsystems/Function-Call Generator  sample_time=-1  numberOfIterations=1
  Resume ISR : Subsystem  TreatAsAtomicUnit=on
  Suspend ISR : Subsystem  TreatAsAtomicUnit=on
  SSCP_pclMotorPowerOrder_SetPowerOrder : Outport
  s16MotorPowerOrder1 : Outport  Port=2
  wires:
  Function-Call Generator/1 -> Demux/1
  Demux/3 -> Resume ISR/Trigger
  Demux/2 -> Call PAL service to update the PWM/Trigger
  Demux/1 -> Suspend ISR/Trigger
  In1/1 -> Call PAL service to update the PWM/1(In1)  "s16MotorPowerOrder"
  Call PAL service to update the PWM/1(SSCP_pclMotorPowerOrder_SetPowerOrder) -> SSCP_pclMotorPowerOrder_SetPowerOrder/1
  Call PAL service to update the PWM/2(s16MotorPowerOrder1) -> s16MotorPowerOrder1/1
  u8MotorStageStatus/1 -> Call PAL service to update the PWM/2(u8MotorStageStatus)

== system BFE_TestHarness/BFE_AC_BeltFunctionExecution/Subsystem/BFE_AC_BeltFunctionExecution/BFE_AC_BeltFunctionExecution/BFE_runExecuteStandardSteps/ExecuteStandardSteps/SubsystemConvertOrderToMotorPower ==
  u8OrderType : Inport  RequirementInfo={} %GIDa_c1767bd6_cb15_4346_873f_f960a3bf96f4
  bIsNewStepBegin : Inport  RequirementInfo={} %GIDa_c3db926f_81b7_4455_a17e_3e049c90ab06  Port=2
  s32OrderToApply : Inport  RequirementInfo={} %GIDa_cf42c4bb_22f2_44b8_bdaa_b199bd1b8048  Port=3
  u16BatteryVoltage : Inport  RequirementInfo={} %GIDa_f3773e77_ee2c_4e4e_8ef8_919075a305d5  Port=4
  u32MeasuredCurrent : Inport  RequirementInfo={} %GIDa_dc07d825_1043_4b65_a4d4_1d0edac69fc3  Port=5
  s8OldPwm : Inport  RequirementInfo={} %GIDa_436bb622_bb55_42dd_b4a9_a2ef53e8ec19  Port=6
  bIsPrevStepHP : Inport  RequirementInfo={} %GIDa_18558ba6_1643_4730_af05_0be4219eff94  Port=7
  Current_Regulation : Subsystem  RequirementInfo={} %GIDa_70967bde_7c32_43e2_b6ba_6c4cfdd379dc  TreatAsAtomicUnit=on
      mask help:
      | Proportional control acts much like a human operator would. The bigger the error, the bigger the actuation applied. This can lead to oscillations or, because of the dynamics, permanent error if the error is not significant enough to create a corrective action. This is called a "steady-state error."
      |
      | Integral control considers the history of the error. It keeps adding the value of the error, consequently removing the steady-state error once the system is near its final state.  In systems with long transitions, however, integral control integrates over time, causing "integral windup," where the system evolves beyond the desired setpoint. The output overshoots " that is, it goes over the desired value before going back and settling. High integral gains may also cause the system to become unstable.
      |
      | Derivative control evolves with the rate of change. This allows the controller to estimate how the error will change in the near future. It makes the system react faster to changes, but it also can make it unstable. Another drawback is that derivatives are very sensitive to noise, making the actuation itself noisy.
  Gain : Gain  RequirementInfo={} %GIDa_cd58ea51_5134_43de_b24a_1216c96f21bd  OutDataTypeStr=uint8  mask(TL_Gain){data={'date',735951.66853343754}}
      settings: CopyFcn=if exist('tl_reset_reviewflag','file')==2,tl_reset_reviewflag(gcbh);end  DeleteFcn=if exist('delete_tlblock','file')==2,delete_tlblock(gcbh);end  NameChangeFcn=if exist('rename_tlblock','file')==2,rename_tlblock(gcbh);end  OpenFcn=if exist('tl_open_blockdlg','file')==2,tl_open_blockdlg(gcbh);else,open_system(gcbh,'parameter');end
      mask Help: eval(['if exist(''tl_online_help'',''file'') == 2, tl_online_help(''Topic'',''TL_Gain''),else, web([''jar:file:///'',matlabroot,''/help/toolbox/simulink/help.jar!/slref/' lower(get_param(gcbh,'Blocktype')) '.html''], ''-helpbrowser''),end'])
      mask Display: plot([0, .9, 0],[.05, .5, .95])
  Init_Error_Calculation : Subsystem  RequirementInfo={} %GIDa_6cf61433_85c4_4853_b431_4af2beb7e94b
  ManageIntegerErrorReset : Subsystem  RequirementInfo={} %GIDa_e14d94ee_8f91_40da_bd18_f3a837e2ce9f  TreatAsAtomicUnit=on
  Merge : Merge  RequirementInfo={} %GIDa_b72214f9_958a_4f06_bc6f_3d38b8a097ca  Inputs=4  InitialOutput=0  mask(TL_Merge){data={'output',{'name','s16UnfilteredMotorCommand','inheritscaling',0},'date',735951.66852557869}}
      settings: CopyFcn=if exist('tl_reset_reviewflag','file')==2,tl_reset_reviewflag(gcbh);end  DeleteFcn=if exist('delete_tlblock','file')==2,delete_tlblock(gcbh);end  NameChangeFcn=if exist('rename_tlblock','file')==2,rename_tlblock(gcbh);end  OpenFcn=if exist('tl_open_blockdlg','file')==2,tl_open_blockdlg(gcbh);else,open_system(gcbh,'parameter');end
      mask Help: eval(['if exist(''tl_online_help'',''file'') == 2, tl_online_help(''Topic'',''TL_Merge''),else, web([''jar:file:///'',matlabroot,''/help/toolbox/simulink/help.jar!/slref/' lower(get_param(gcbh,'Blocktype')) '.html''], ''-helpbrowser''),end'])
      mask Display: plot([-0.05, 1.05, NaN, -0.05, 1.05],[.01, .01, NaN, .99, .99])
  MotorVoltage_Regulation : Subsystem  RequirementInfo={} %GIDa_7f07ea4e_d245_4c2e_81d3_d72628b54a8a  TreatAsAtomicUnit=on
  No_Regulation : Subsystem  RequirementInfo={} %GIDa_d5a3b940_13e2_4ede_a354_2ed1535a0596  TreatAsAtomicUnit=on
  PWM_Regulation : Subsystem  RequirementInfo={} %GIDa_34f9cb08_cb2a_427a_91c4_ba42591d05fa  TreatAsAtomicUnit=on
  RescaleOrderType : Subsystem  RequirementInfo={} %GIDa_ef2ab81f_5afa_40b0_8ba8_f176ab08f51d  TreatAsAtomicUnit=on
  SwitchCase : SwitchCase  RequirementInfo={} %GIDa_e18c9de3_2555_49d8_bf48_d7ed55334f23  CaseConditions={0,1,4}
  Unit Delay : UnitDelay  RequirementInfo={} %GIDa_d1526458_66fe_4074_9458_9a5c5fb4c80a  SampleTime=-1  mask(TL_UnitDelay){data={'output',{'type','Int32'},'state',{'name','X_s32OldInteger','type','Int32'},'date',735951.66850642359}}
      settings: CopyFcn=if exist('tl_reset_reviewflag','file')==2,tl_reset_reviewflag(gcbh);end  DeleteFcn=if exist('delete_tlblock','file')==2,delete_tlblock(gcbh);end  NameChangeFcn=if exist('rename_tlblock','file')==2,rename_tlblock(gcbh);end  OpenFcn=if exist('tl_open_blockdlg','file')==2,tl_open_blockdlg(gcbh);else,open_system(gcbh,'parameter');end
      mask Help: eval(['if exist(''tl_online_help'',''file'') == 2, tl_online_help(''Topic'',''TL_UnitDelay''),else, web([''jar:file:///'',matlabroot,''/help/toolbox/simulink/help.jar!/slref/' lower(get_param(gcbh,'Blocktype')) '.html''], ''-helpbrowser''),end'])
      mask Display: plot([-0.05, 1.05, NaN, -0.05, 1.05],[.01, .01, NaN, .99, .99])
  Unit Delay1 : UnitDelay  RequirementInfo={} %GIDa_c4de7eb0_e0d7_4780_9fb8_899132ed6865  SampleTime=-1  mask(TL_UnitDelay){data={'output',{'type','Bool'},'state',{'name','bIsNewCycle2ms','type','Bool'},'date',735951.66850587958}}
      settings: CopyFcn=if exist('tl_reset_reviewflag','file')==2,tl_reset_reviewflag(gcbh);end  DeleteFcn=if exist('delete_tlblock','file')==2,delete_tlblock(gcbh);end  NameChangeFcn=if exist('rename_tlblock','file')==2,rename_tlblock(gcbh);end  OpenFcn=if exist('tl_open_blockdlg','file')==2,tl_open_blockdlg(gcbh);else,open_system(gcbh,'parameter');end
      mask Help: eval(['if exist(''tl_online_help'',''file'') == 2, tl_online_help(''Topic'',''TL_UnitDelay''),else, web([''jar:file:///'',matlabroot,''/help/toolbox/simulink/help.jar!/slref/' lower(get_param(gcbh,'Blocktype')) '.html''], ''-helpbrowser''),end'])
      mask Display: plot([-0.05, 1.05, NaN, -0.05, 1.05],[.01, .01, NaN, .99, .99])
  s16UnsaturatedMotorPower : Outport  RequirementInfo={} %GIDa_230bb7a4_30fd_4050_8455_804c66798185
  wires:
  u16BatteryVoltage/1 -> MotorVoltage_Regulation/2(usBatteryVoltage), Current_Regulation/4(u16BatteryVoltage)  "u16BatteryVoltage"
  PWM_Regulation/1(s16Consign) -> Merge/1
  SwitchCase/4 -> No_Regulation/Action
  SwitchCase/1 -> PWM_Regulation/Action
  Merge/1 -> s16UnsaturatedMotorPower/1  "sUnsaturatedMotorPower"
  s32OrderToApply/1 -> PWM_Regulation/1(s32OrderToApply), MotorVoltage_Regulation/1(lOrderToApply), Current_Regulation/1(s32OrderToApply)  "s32OrderToApply"
  MotorVoltage_Regulation/1(sUnsaturatedMotorPowerOrder) -> Merge/3
  No_Regulation/1(s16Consign) -> Merge/4
  u8OrderType/1 -> RescaleOrderType/1(u8OrderType), ManageIntegerErrorReset/1(u8OrderType)
  RescaleOrderType/1(OrderType_Rescaled) -> Gain/1
  SwitchCase/3 -> MotorVoltage_Regulation/Action
  Current_Regulation/1(s16UnsaturatedMoterPowerOrder) -> Merge/2
  SwitchCase/2 -> Current_Regulation/Action
  u32MeasuredCurrent/1 -> Current_Regulation/2(u32MeasuredCurrent)
  s8OldPwm/1 -> Init_Error_Calculation/2(s8OldPWM), Current_Regulation/3(s16OldPWM)
  RescaleOrderType/3(IsPID_S) -> Current_Regulation/7(bIsPIDSupply)
  RescaleOrderType/2(bIsPID_M) -> Current_Regulation/6(bIsPIDMotor)
  Gain/1 -> SwitchCase/1
  ManageIntegerErrorReset/2(b8IsNewCycle) -> Unit Delay1/1
  Unit Delay1/1 -> Current_Regulation/5(bIsNewCycle)
  bIsNewStepBegin/1 -> Current_Regulation/9(bIsNewStepBegin)
  ManageIntegerErrorReset/1(s32OldErrorFiltered) -> Unit Delay/1
  Current_Regulation/2(s32IntegerError) -> ManageIntegerErrorReset/2(s32IntegerErrorBeforeFiltering)
  bIsPrevStepHP/1 -> Init_Error_Calculation/1(bIsPRevStepHP)
  Unit Delay/1 -> Init_Error_Calculation/3(s32OldErrorInteger)
  Init_Error_Calculation/1(s32OldErrorIntegerOut) -> Current_Regulation/8(s32OldErrorInteger)
